simulink model "PMSM_model_og_tf_med_kv"  (R2015b)
settings: Solver=VariableStepAuto  StartTime=0.0  StopTime=10.0  RelTol=1e-3
values from neighbouring files (symbols this model uses):
  J_pro = (m*r^2+J_G2)*(G1/G2)^2 + J_G1    (= 0.281547798877)    [Control_Parameters.m]    (also in M_fil_til_jacob.m; PMSM_State_Space_Parameters.m)
  Kt = .07329    (= 0.07329)    [Control_Parameters.m]    (also in M_fil_til_jacob.m; PMSM_State_Space_Parameters.m)
  Kv = 0.001    [Control_Parameters.m]    (also in M_fil_til_jacob.m)
  L = 4e-5    (= 4e-05)    [Control_Parameters.m]    (also in M_fil_til_jacob.m; PMSM_State_Space_Parameters.m)
  R = .013/2    (= 0.0065)    [Control_Parameters.m]    (also in M_fil_til_jacob.m; PMSM_State_Space_Parameters.m)
undefined symbols (not defined in the file or in its folder): sigbuilder_block
libraries: simulink x1
settings Model: Creator=Morten  LastModifiedBy=Morten

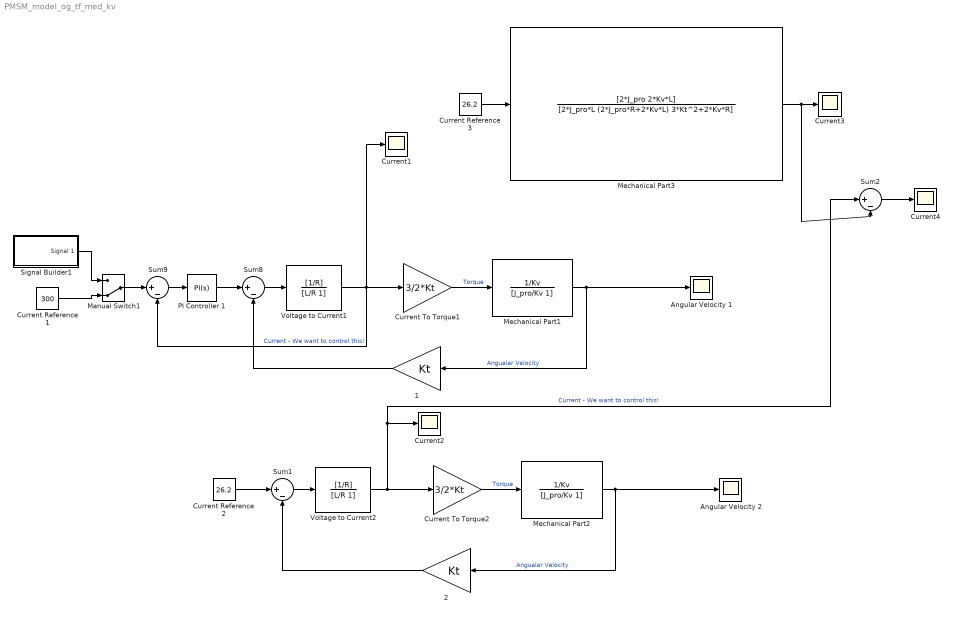
== system PMSM_model_og_tf_med_kv ==
  "             1" : Gain  Gain=Kt
  "             2" : Gain  Gain=Kt
  Angular Velocity 1 : Scope
  Angular Velocity 2 : Scope
  Current Reference 1 : Constant  Value=300
  Current Reference 2 : Constant  Value=26.2
  Current Reference 3 : Constant  Value=26.2
  Current To Torque1 : Gain  Gain=3/2*Kt
  Current To Torque2 : Gain  Gain=3/2*Kt
  Current{1..4} (4 alike) : Scope
  Manual Switch1 : ManualSwitch  CurrentSetting=0
  Mechanical Part1 : TransferFcn  Numerator=1/Kv  Denominator=[J_pro/Kv 1]
  Mechanical Part2 : TransferFcn  Numerator=1/Kv  Denominator=[J_pro/Kv 1]
  Mechanical Part3 : TransferFcn  Numerator=[2*J_pro 2*Kv*L]  Denominator=[2*J_pro*L (2*J_pro*R+2*Kv*L) 3*Kt^2+2*Kv*R]
  PI Controller 1 : simulink/Continuous/PID Controller  Controller=PI  TimeDomain=Continuous-time  SampleTime=-1  IntegratorMethod=Forward Euler  FilterMethod=Forward Euler  Form=Parallel  UseFilter=on  ControllerParametersSource=internal  P=0.0522182495496133  I=8.48921468617953  D=0  N=100  InitialConditionSource=internal  InitialConditionForIntegrator=0  InitialConditionForFilter=0  ExternalReset=none  LimitOutput=off  UpperSaturationLimit=inf  LowerSaturationLimit=-inf  LinearizeAsGain=on  AntiWindupMode=none  Kb=1  TrackingMode=off  Kt=1  PParamMin=[]  PParamMax=[]  IParamMin=[]  IParamMax=[]  DParamMin=[]  DParamMax=[]  NParamMin=[]  NParamMax=[]  KbParamMin=[]  KbParamMax=[]  KtParamMin=[]  KtParamMax=[]  POutMin=[]  POutMax=[]  IOutMin=[]  IOutMax=[]  DOutMin=[]  DOutMax=[]  NOutMin=[]  NOutMax=[]  KbOutMin=[]  KbOutMax=[]  KtOutMin=[]  KtOutMax=[]  IntegratorOutMin=[]  IntegratorOutMax=[]  FilterOutMin=[]  FilterOutMax=[]  SumOutMin=[]  SumOutMax=[]  SumI1OutMin=[]  SumI1OutMax=[]  SumI2OutMin=[]  SumI2OutMax=[]  SumI3OutMin=[]  SumI3OutMax=[]  SumDOutMin=[]  SumDOutMax=[]  SaturationOutMin=[]  SaturationOutMax=[]  IntegratorContinuousStateAttributes=''  IntegratorStateMustResolveToSignalObject=off  IntegratorRTWStateStorageClass=Auto  FilterContinuousStateAttributes=''  FilterStateMustResolveToSignalObject=off  FilterRTWStateStorageClass=Auto  DifferentiatorICPrevScaledInput=0  DifferentiatorOutMin=[]  DifferentiatorOutMax=[]
  Signal Builder1 : Subsystem  Tag=STV Subsys  LoadFcn=sigbuilder_block('load');  StartFcn=sigbuilder_block('start');  StopFcn=sigbuilder_block('stop');  ClipboardFcn=sigbuilder_block('clipboard');  mask(Sigbuilder block){}
      mask help: Simulink:masks:SigbuilderBlock_MD
      mask init:
      | if ~strcmp(get_param(bdroot(gcbh),'SimulationStatus'),'stopped') tuvar = sigbuilder_block('maskInit'); end
      settings: CopyFcn=sigbuilder_block('copy');  DeleteFcn=sigbuilder_block('delete');  ModelCloseFcn=sigbuilder_block('modelClose');  PreSaveFcn=sigbuilder_block('preSave');  PauseFcn=sigbuilder_block('pause');  ContinueFcn=sigbuilder_block('continue');  NameChangeFcn=sigbuilder_block('namechange');  OpenFcn=sigbuilder_block('open',[437.6 199.2 550.4 400 ]);  CloseFcn=sigbuilder_block('close');
      mask Display: plot(0, 0, 100, 100,[2, 2, 32, 32, 2], [68, 8, 8, 68, 68],[32, 2], [38, 38], [32, 19, 2],[53, 60, 44], [32, 17, 17, 2],[16, 16, 31, 31]);txt = getActiveGroup(gcbh);text(2, 100, txt,'verticalAlignment', 'top');
  Sum{1..2,8..9} (4 alike) : Sum  Inputs=|+-
  Voltage to Current1 : TransferFcn  Numerator=[1/R]  Denominator=[L/R 1]
  Voltage to Current2 : TransferFcn  Numerator=[1/R]  Denominator=[L/R 1]
  wires:
  "             1"/1 -> Sum8/2
  Sum8/1 -> Voltage to Current1/1
  Voltage to Current1/1 -> Current1/1, Current To Torque1/1, Sum9/2  "Current - We want to control this!"
  Current To Torque1/1 -> Mechanical Part1/1  "Torque"
  PI Controller 1/1 -> Sum8/1
  Sum9/1 -> PI Controller 1/1
  Signal Builder1/1(Signal 1) -> Manual Switch1/1
  Mechanical Part1/1 -> "             1"/1, Angular Velocity 1/1  "Angualar Velocity"
  Current Reference 1/1 -> Manual Switch1/2
  Manual Switch1/1 -> Sum9/1
  "             2"/1 -> Sum1/2
  Sum1/1 -> Voltage to Current2/1
  Voltage to Current2/1 -> Sum2/1, Current2/1, Current To Torque2/1  "Current - We want to control this!"
  Current To Torque2/1 -> Mechanical Part2/1  "Torque"
  Current Reference 2/1 -> Sum1/1
  Mechanical Part2/1 -> Angular Velocity 2/1, "             2"/1  "Angualar Velocity"
  ? -> ?
  Mechanical Part3/1 -> Sum2/2, Current3/1
  Current Reference 3/1 -> Mechanical Part3/1
  Sum2/1 -> Current4/1

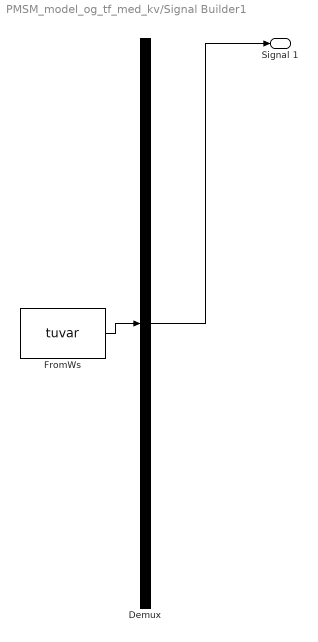
== system PMSM_model_og_tf_med_kv/Signal Builder1 ==
  Demux : Demux  Tag=STV Demux  Outputs=1
  FromWs : FromWorkspace  Tag=STV FromWs  VariableName=tuvar  SampleTime=0
      SigBuilderData=|
      | common.afterFinalStr = 'Extrapolate'
      | common.sampleTime = 0
      | dataSet.timeRange = [0 10]
      | dataSet.name = 'Group 1'
      | sbobj.Groups.Name = 'Group 1'
      | sbobj.Groups.Signals.Name = 'Signal 1'
      | sbobj.Groups.Signals.XData = [0 0.1 4 6 6 10]
      | sbobj.Groups.Signals.YData = [0 300 300 1 0 0]
  Signal 1 : Outport  Tag=STV Outport
  wires:
  Demux/1 -> Signal 1/1
  FromWs/1 -> Demux/1
